simulink model "quarter_sus_imp"  (R2025a)
settings: Solver=FixedStepAuto  StartTime=0.0  StopTime=20  FixedStep=0.001  RelTol=1e-3
model workspace (MAT data in the model file):
  Cs : Simulink.Parameter (value not decoded)
  Cy_f1 = 128915.5
  Cy_r1 = 85943.6
  G0 : Simulink.Parameter (value not decoded)
  IDA_ISD_PBC_bd : Simulink.Parameter (value not decoded)
  IDA_ISD_PBC_c1 : Simulink.Parameter (value not decoded)
  IDA_ISD_PBC_k1 : Simulink.Parameter (value not decoded)
  IDA_ISD_PBC_k2 : Simulink.Parameter (value not decoded)
  IDA_ISD_PBC_r1 : Simulink.Parameter (value not decoded)
  IDA_PBC_cd4 = 2000
  IDA_PBC_kd2 = 10000
  IDA_PBC_r1 = 1.5
  IDA_PBC_r2 = 0.44
  ISD_1_b : Simulink.Parameter (value not decoded)
  ISD_1_c : Simulink.Parameter (value not decoded)
  ISD_1_k1 : Simulink.Parameter (value not decoded)
  ISD_1_k2 : Simulink.Parameter (value not decoded)
  Izz1 = 1536.7
  Ks : Simulink.Parameter (value not decoded)
  Kt : Simulink.Parameter (value not decoded)
  Q : Simulink.Parameter (value not decoded)
  Q_dot : Simulink.Parameter (value not decoded)
  Q_dot_s : Simulink.Parameter (value not decoded)
  Q_dot_u : Simulink.Parameter (value not decoded)
  Q_flec : Simulink.Parameter (value not decoded)
  SHADD_alpha : Simulink.Parameter (value not decoded)
  a1 = 1.015
  a_max : Simulink.Parameter (value not decoded)
  a_min : Simulink.Parameter (value not decoded)
  adva_max : Simulink.Parameter (value not decoded)
  adva_min : Simulink.Parameter (value not decoded)
  as_max : Simulink.Parameter (value not decoded)
  b1 = 1.895
  b_deflec : Simulink.Parameter (value not decoded)
  bump_height : Simulink.Parameter (value not decoded)
  bump_lenth : Simulink.Parameter (value not decoded)
  bump_start : Simulink.Parameter (value not decoded)
  damper_param : Simulink.Parameter (value not decoded)
  deflec_max : Simulink.Parameter (value not decoded)
  done_range : Simulink.Parameter (value not decoded)
  f0 : Simulink.Parameter (value not decoded)
  h1 = 0.54
  imp_Cs : Simulink.Parameter (value not decoded)
  imp_Ks : Simulink.Parameter (value not decoded)
  imp_Ms : Simulink.Parameter (value not decoded)
  inerter_b : Simulink.Parameter (value not decoded)
  inerter_b_2 : Simulink.Parameter (value not decoded)
  inerter_c : Simulink.Parameter (value not decoded)
  inerter_k : Simulink.Parameter (value not decoded)
  inerter_k_2 : Simulink.Parameter (value not decoded)
  ms : Simulink.Parameter (value not decoded)
  mu : Simulink.Parameter (value not decoded)
  noise_seed : Simulink.Parameter (value not decoded)
  punish_Q : Simulink.Parameter (value not decoded)
  punish_R : Simulink.Parameter (value not decoded)
  reward_w_as : Simulink.Parameter (value not decoded)
  reward_w_au : Simulink.Parameter (value not decoded)
  reward_w_defv : Simulink.Parameter (value not decoded)
  road_seed : Simulink.Parameter (value not decoded)
  road_type : Simulink.Parameter (value not decoded)
  sigma_f1 = 0.1
  sigma_r1 = 0.1
  sine_amp : Simulink.Parameter (value not decoded)
  sine_freq : Simulink.Parameter (value not decoded)
  u : Simulink.Parameter (value not decoded)
  vs0 : Simulink.Parameter (value not decoded)
  vu0 : Simulink.Parameter (value not decoded)
  x_max : Simulink.Parameter (value not decoded)
  x_min : Simulink.Parameter (value not decoded)
  xs0 : Simulink.Parameter (value not decoded)
  xu0 : Simulink.Parameter (value not decoded)
symbols that are objects in the model workspace (value not decoded): a_max, a_min, b_deflec, bump_height, bump_lenth, bump_start, Cs, damper_param, f0, G0, IDA_ISD_PBC_bd, IDA_ISD_PBC_c1, IDA_ISD_PBC_k1, IDA_ISD_PBC_k2, IDA_ISD_PBC_r1, imp_Cs, imp_Ks, imp_Ms, Ks, Kt, ms, mu, Q_dot_s, Q_dot_u, Q_flec, road_type, SHADD_alpha, sine_amp, sine_freq, vs0, vu0, xs0, xu0
undefined symbols (not defined in the file or in its folder): ADD, Force, IDA, Imp, PBC, SH, Train, Validation
libraries: fl_lib x32, nesl_utility x27, sdl_lib x2, deeplib x1, simulink x1
(part 4 of 5)

== system quarter_sus_imp/QuarterSuspension /road_profile/origin ==
  Manual Switch : ManualSwitch  CurrentSetting=0
  Radio Button : RadioButtonGroup  LabelPosition=Hide  SelectedLabel=随机路面  ButtonGroupName=Group
  Road_Type : Constant  Value=road_type  OutDataTypeStr=int8
  road_profile : Subsystem
  路面选择 : Constant  Value=3  OutDataTypeStr=int8
  "Road " : Outport
  wires:
  路面选择/1 -> Manual Switch/1
  road_profile/1("Road ") -> "Road "/1  "Zr"
  Manual Switch/1 -> road_profile/1(Road_selection)
  Road_Type/1 -> Manual Switch/2

== system quarter_sus_imp/QuarterSuspension /Subsystem1/Active Suspension/Subsystem ==
  Connection Port : PMIOPort  Side=Left

== system quarter_sus_imp/QuarterSuspension /Subsystem1/Semi Active Air Suspension/Damper ==
  displacement : Inport
  velocity : Inport  Port=2
  current : Inport  Port=3
  Hysteretic : Subsystem  VariantControl=Hysteretic
  Linear : Subsystem  VariantControl=simple linear
  Random Current : Subsystem  VariantControl=Random Current
  semi-active : Subsystem  VariantControl=Semi-active
  simple_Nonlinear : Subsystem  VariantControl=Simple_Nonlinear
  simple_Nonlinear_2d : Subsystem  VariantControl=Simple_Nonlinear_2d
  F_d : Outport
  current_log : Outport  Port=2

== system quarter_sus_imp/QuarterSuspension /Subsystem1/Semi Active Air Suspension/Subsystem ==
  In1 : Inport
  linear : Subsystem  VariantControl=linear
  simple nonlinear : Subsystem  VariantControl=simple nonlinear
  Out1 : Outport

== system quarter_sus_imp/QuarterSuspension /Subsystem1/Semi Active Air Suspension simscape/Damper ==
  displacement : Inport
  velocity : Inport  Port=2
  current : Inport  Port=3
  Hysteretic : Subsystem  VariantControl=Hysteretic
  Random Current : Subsystem  VariantControl=Random Current
  semi-active : Subsystem  VariantControl=Semi-active
  simple_Nonlinear : Subsystem  VariantControl=Simple_Nonlinear
  simple_Nonlinear_2d : Subsystem  VariantControl=Simple_Nonlinear_2d
  F_d : Outport
  current_log : Outport  Port=2

== system quarter_sus_imp/QuarterSuspension /Subsystem1/Semi Active Air Suspension simscape/Subsystem ==
  Connection Port : PMIOPort  Side=Left

== system quarter_sus_imp/QuarterSuspension /Subsystem1/Semi Active Suspension/Damper ==
  displacement : Inport
  velocity : Inport  Port=2
  current : Inport  Port=3
  Hysteretic : Subsystem  VariantControl=Hysteretic
  Random Current : Subsystem  VariantControl=Random Current
  semi-active : Subsystem  VariantControl=Semi-active
  simple_Nonlinear : Subsystem  VariantControl=Simple_Nonlinear
  simple_Nonlinear_2d : Subsystem  VariantControl=Simple_Nonlinear_2d
  F_d : Outport
  current_log : Outport  Port=2

== system quarter_sus_imp/QuarterSuspension /Variant Subsystem/ADD/Subsystem1 ==
  state : Inport
  Demux : Demux  Outputs=11
  Divide : Product  Inputs=**
  Switch1 : Switch  SaturateOnIntegerOverflow=off  InputSameDT=off
  Terminator{,1..6} (7 alike) : Terminator
  c_max : Constant  Value=500
  c_min : Constant  Value=-500
  action : Outport
  wires:
  state/1 -> Demux/1
  Demux/10 -> Terminator2/1
  Demux/7 -> [v_deflection]
  Demux/11 -> Terminator3/1
  Demux/6 -> [deflection]
  Demux/3 -> [as]
  Demux/2 -> [vs]
  Demux/1 -> Terminator6/1
  Demux/5 -> Terminator5/1
  Demux/4 -> Terminator4/1
  Demux/8 -> Terminator/1
  Demux/9 -> Terminator1/1
  c_min/1 -> Switch1/3
  Divide/1 -> Switch1/2
  c_max/1 -> Switch1/1
  [as] -> Divide/1
  [v_deflection] -> Divide/2
  Switch1/1 -> action/1

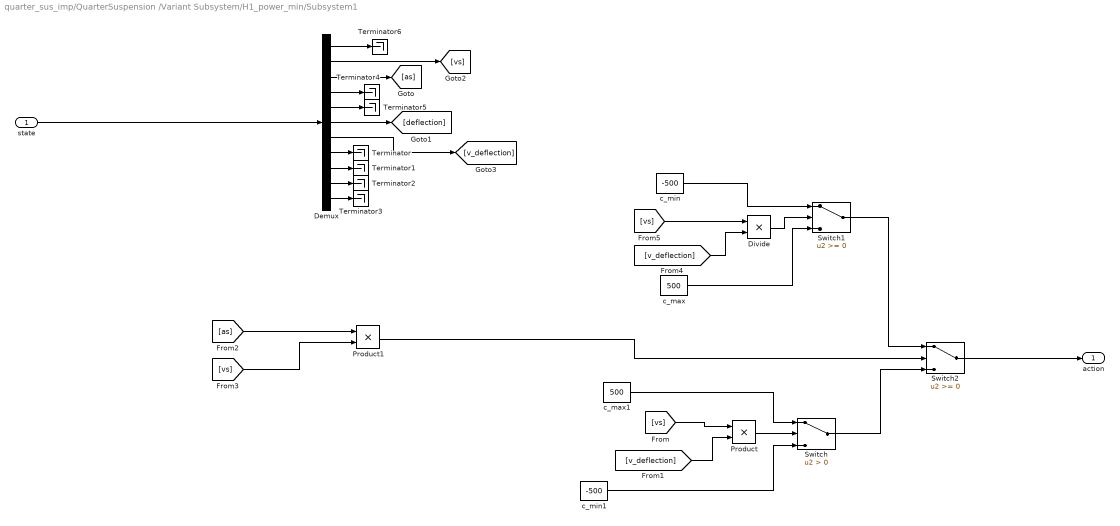
== system quarter_sus_imp/QuarterSuspension /Variant Subsystem/H1_power_min/Subsystem1 ==
  state : Inport
  Demux : Demux  Outputs=11
  Divide : Product  Inputs=**
  Product : Product
  Product1 : Product
  Switch : Switch  Criteria=u2 > Threshold  SaturateOnIntegerOverflow=off  InputSameDT=off
  Switch1 : Switch  SaturateOnIntegerOverflow=off  InputSameDT=off
  Switch2 : Switch  SaturateOnIntegerOverflow=off  InputSameDT=off
  Terminator{,1..6} (7 alike) : Terminator
  c_max : Constant  Value=500
  c_max1 : Constant  Value=500
  c_min : Constant  Value=-500
  c_min1 : Constant  Value=-500
  action : Outport
  wires:
  state/1 -> Demux/1
  Demux/10 -> Terminator2/1
  Demux/7 -> [v_deflection]
  Demux/11 -> Terminator3/1
  Demux/6 -> [deflection]
  Demux/3 -> [as]
  Demux/2 -> [vs]
  Demux/1 -> Terminator6/1
  Demux/5 -> Terminator5/1
  Demux/4 -> Terminator4/1
  Demux/8 -> Terminator/1
  Demux/9 -> Terminator1/1
  c_min/1 -> Switch1/1
  Divide/1 -> Switch1/2
  c_max/1 -> Switch1/3
  [vs] -> Divide/1
  [v_deflection] -> Divide/2
  c_min1/1 -> Switch/3
  Product/1 -> Switch/2
  [v_deflection] -> Product/2
  c_max1/1 -> Switch/1
  [vs] -> Product/1
  [vs] -> Product1/2
  Product1/1 -> Switch2/2
  Switch2/1 -> action/1
  Switch/1 -> Switch2/3
  Switch1/1 -> Switch2/1
  [as] -> Product1/1

== system quarter_sus_imp/QuarterSuspension /Variant Subsystem/IDA-PBC/Subsystem ==
  In1 : Inport
  IDA-PBC 论文控制 : Subsystem  VariantControl=IDAPBC
  IDA_ISD_1号参考控制 : Subsystem  VariantControl=My_IDA_ISD
  我的控制 : Subsystem  VariantControl=MyIDA_PBC
  u : Outport

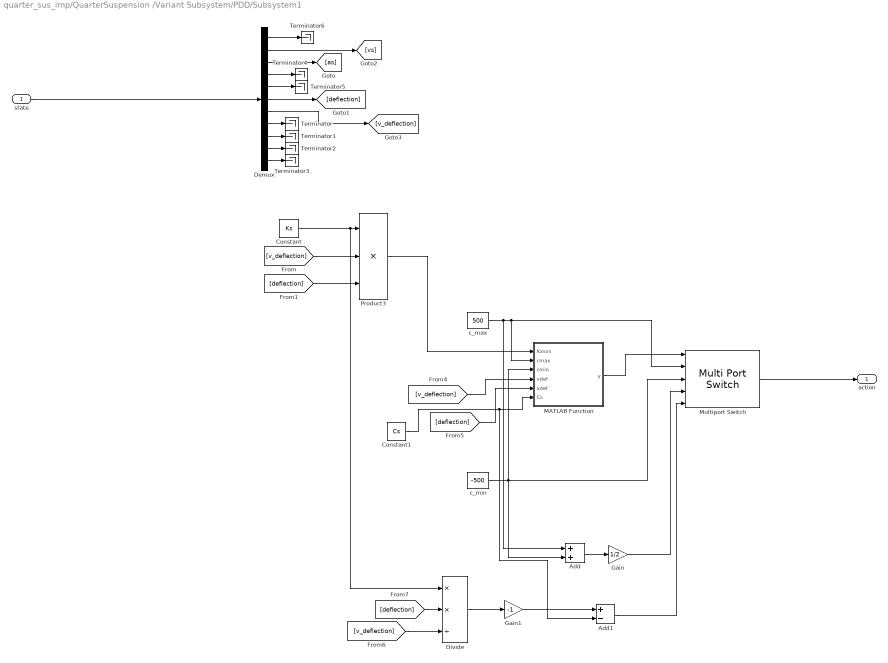
== system quarter_sus_imp/QuarterSuspension /Variant Subsystem/PDD/Subsystem1 ==
  state : Inport
  Add : Sum
  Add1 : Sum  Inputs=+-
  Constant : Constant  Value=Ks
  Constant1 : Constant  Value=Cs
  Demux : Demux  Outputs=11
  Divide : Product  Inputs=**/
  Gain : Gain  Gain=1/2
  Gain1 : Gain  Gain=-1
  MATLAB Function : MATLAB Function  TreatAsAtomicUnit=on
  Multiport Switch : MultiPortSwitch  Inputs=4  SaturateOnIntegerOverflow=off  InputSameDT=off
  Product3 : Product  Inputs=3
  Terminator{,1..6} (7 alike) : Terminator
  c_max : Constant  Value=500
  c_min : Constant  Value=-500
  action : Outport
  wires:
  state/1 -> Demux/1
  Demux/10 -> Terminator2/1
  Demux/7 -> [v_deflection]
  Demux/11 -> Terminator3/1
  Demux/6 -> [deflection]
  Demux/3 -> [as]
  Demux/2 -> [vs]
  Demux/1 -> Terminator6/1
  Demux/5 -> Terminator5/1
  Demux/4 -> Terminator4/1
  Demux/8 -> Terminator/1
  Demux/9 -> Terminator1/1
  c_max/1 -> Multiport Switch/2, MATLAB Function/2(cmax), Add/1
  Multiport Switch/1 -> action/1
  Constant/1 -> Divide/1, Product3/1
  [v_deflection] -> Product3/2
  [deflection] -> Product3/3
  Product3/1 -> MATLAB Function/1(Kxsvs)
  c_min/1 -> Multiport Switch/3, Add/2, MATLAB Function/3(cmin)
  MATLAB Function/1(y) -> Multiport Switch/1
  [v_deflection] -> MATLAB Function/4(vdef)
  Add/1 -> Gain/1
  [deflection] -> MATLAB Function/5(xdef)
  [v_deflection] -> Divide/3
  [deflection] -> Divide/2
  Divide/1 -> Gain1/1
  Gain/1 -> Multiport Switch/4
  Add1/1 -> Multiport Switch/5
  Constant1/1 -> MATLAB Function/6(Cs), Add1/2
  Gain1/1 -> Add1/1

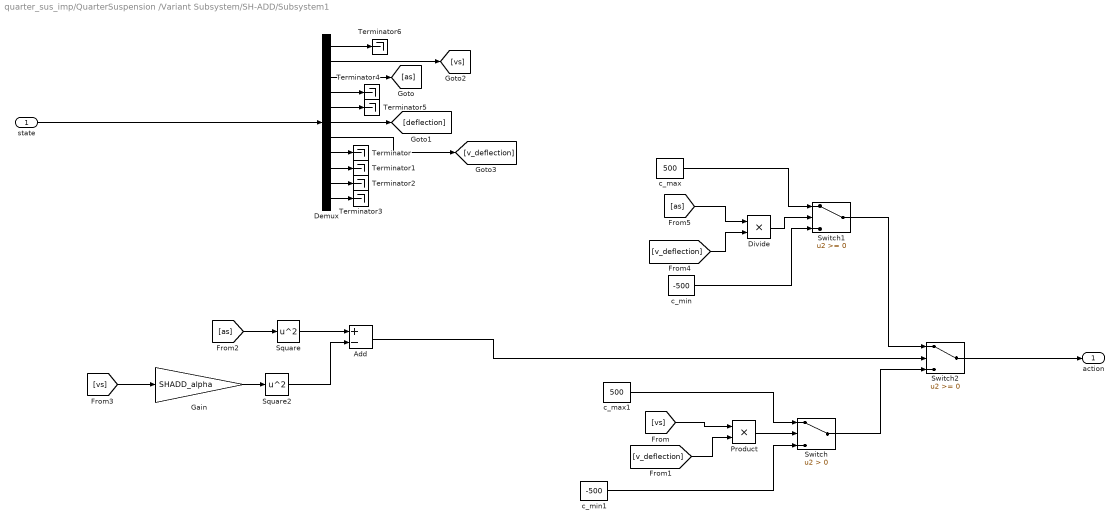
== system quarter_sus_imp/QuarterSuspension /Variant Subsystem/SH-ADD/Subsystem1 ==
  state : Inport
  Add : Sum  Inputs=+-
  Demux : Demux  Outputs=11
  Divide : Product  Inputs=**
  Gain : Gain  Gain=SHADD_alpha
  Product : Product
  Square : Math  Operator=square
  Square2 : Math  Operator=square
  Switch : Switch  Criteria=u2 > Threshold  SaturateOnIntegerOverflow=off  InputSameDT=off
  Switch1 : Switch  SaturateOnIntegerOverflow=off  InputSameDT=off
  Switch2 : Switch  SaturateOnIntegerOverflow=off  InputSameDT=off
  Terminator{,1..6} (7 alike) : Terminator
  c_max : Constant  Value=500
  c_max1 : Constant  Value=500
  c_min : Constant  Value=-500
  c_min1 : Constant  Value=-500
  action : Outport
  wires:
  state/1 -> Demux/1
  Demux/10 -> Terminator2/1
  Demux/7 -> [v_deflection]
  Demux/11 -> Terminator3/1
  Demux/6 -> [deflection]
  Demux/3 -> [as]
  Demux/2 -> [vs]
  Demux/1 -> Terminator6/1
  Demux/5 -> Terminator5/1
  Demux/4 -> Terminator4/1
  Demux/8 -> Terminator/1
  Demux/9 -> Terminator1/1
  c_min/1 -> Switch1/3
  Divide/1 -> Switch1/2
  c_max/1 -> Switch1/1
  [as] -> Divide/1
  [v_deflection] -> Divide/2
  c_min1/1 -> Switch/3
  Product/1 -> Switch/2
  [v_deflection] -> Product/2
  c_max1/1 -> Switch/1
  [vs] -> Product/1
  [as] -> Square/1
  [vs] -> Gain/1
  Square/1 -> Add/1
  Gain/1 -> Square2/1
  Add/1 -> Switch2/2
  Switch2/1 -> action/1
  Switch/1 -> Switch2/3
  Switch1/1 -> Switch2/1
  Square2/1 -> Add/2

== system quarter_sus_imp/QuarterSuspension /Variant Subsystem/Skyhook/Subsystem ==
  In1 : Inport
  Add : Sum  Inputs=+-
  Add1 : Sum  Inputs=+-
  Demux : Demux
  Product : Product
  Switch : Switch  Criteria=u2 > Threshold  SaturateOnIntegerOverflow=off  InputSameDT=off
  c_max : Constant  Value=0.9
  c_min : Constant  Value=0.3
  Out8 : Outport
  wires:
  In1/1 -> Demux/1
  c_min/1 -> Switch/3
  Add1/1 -> [v_deflection]
  Add/1 -> [deflection]
  [vs] -> Product/1
  c_max/1 -> Switch/1
  [v_deflection] -> Product/2
  Product/1 -> Switch/2
  Switch/1 -> Out8/1
  Demux/1 -> Add/1
  Demux/2 -> Add/2
  Demux/3 -> Add1/1
  Demux/4 -> Add1/2

== system quarter_sus_imp/QuarterSuspension /Variant Subsystem/Vaildation-3para-feedback/Impedance Controller ==
  feedback_para : Inport
  est_state : Inport  Port=2
  Add1 : Sum  Inputs=+++
  Demux : Demux  Outputs=3
  Demux2 : Demux  Outputs=5
  Product : Product
  Product2 : Product
  Product3 : Product
  F_imp : Outport
  wires:
  Demux/3 -> [feedback_C]
  Demux/1 -> [feedback_M]
  feedback_para/1 -> Demux/1
  Demux/2 -> [feedback_K]
  est_state/1 -> Demux2/1
  Demux2/1 -> [est_Xs]
  Demux2/2 -> [est_Vs]
  Demux2/4 -> [est_Xdef]
  Demux2/5 -> [est_V_def]
  [est_Vs] -> Product2/2
  [feedback_C] -> Product2/1
  [feedback_K] -> Product3/1
  [est_Xs] -> Product3/2
  Product2/1 -> Add1/1
  Product3/1 -> Add1/2
  Add1/1 -> F_imp/1
  [feedback_M] -> Product/2
  Demux2/3 -> [est_as]
  [est_as] -> Product/1
  Product/1 -> Add1/3

== system quarter_sus_imp/QuarterSuspension /Variant Subsystem/Vaildation-3para-feedback/Subsystem ==
  In1 : Inport
  GOPS_Bridge : Subsystem  VariantControl=GOPS_Bridge
  ONNX : Subsystem  VariantControl=ONNX
  real_act : Outport

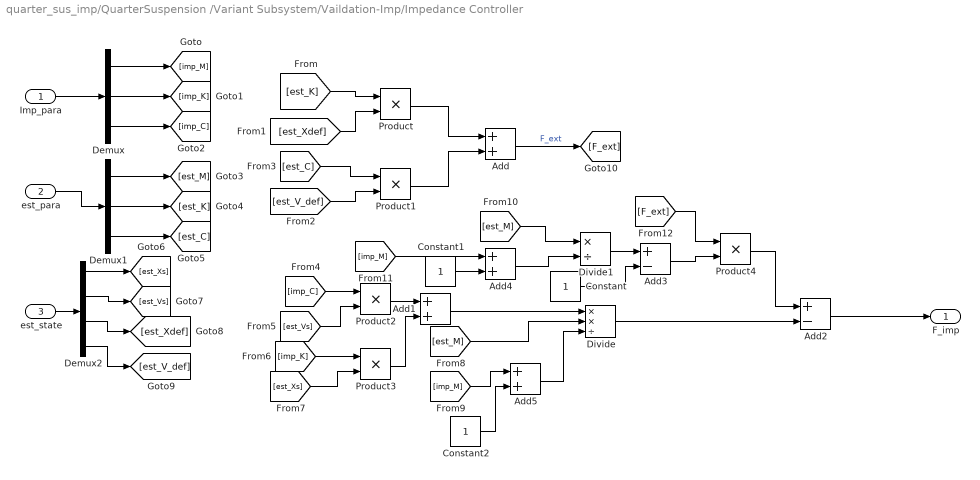
== system quarter_sus_imp/QuarterSuspension /Variant Subsystem/Vaildation-Imp/Impedance Controller ==
  Imp_para : Inport
  est_para : Inport  Port=2
  est_state : Inport  Port=3
  Add{,1,4..5} (4 alike) : Sum
  Add2 : Sum  Inputs=+-
  Add3 : Sum  Inputs=+-
  Constant : Constant
  Constant1 : Constant
  Constant2 : Constant
  Demux : Demux  Outputs=3
  Demux1 : Demux  Outputs=3
  Demux2 : Demux
  Divide : Product  Inputs=**/
  Divide1 : Product  Inputs=*/
  Product{,1..4} (5 alike) : Product
  F_imp : Outport
  wires:
  Demux/3 -> [imp_C]
  Demux/1 -> [imp_M]
  Imp_para/1 -> Demux/1
  Demux/2 -> [imp_K]
  Demux1/1 -> [est_M]
  Demux1/2 -> [est_K]
  est_para/1 -> Demux1/1
  Demux1/3 -> [est_C]
  est_state/1 -> Demux2/1
  Demux2/1 -> [est_Xs]
  Demux2/2 -> [est_Vs]
  Demux2/3 -> [est_Xdef]
  Demux2/4 -> [est_V_def]
  [est_K] -> Product/1
  [est_Xdef] -> Product/2
  [est_C] -> Product1/1
  [est_V_def] -> Product1/2
  Product/1 -> Add/1
  Product1/1 -> Add/2
  Add/1 -> [F_ext]  "F_ext"
  [est_Vs] -> Product2/2
  [imp_C] -> Product2/1
  [imp_K] -> Product3/1
  [est_Xs] -> Product3/2
  Product2/1 -> Add1/1
  Product3/1 -> Add1/2
  Add1/1 -> Divide/1
  [est_M] -> Divide/2
  [imp_M] -> Add5/1
  Divide/1 -> Add2/2
  Add2/1 -> F_imp/1
  [imp_M] -> Add4/1
  [est_M] -> Divide1/1
  Divide1/1 -> Add3/1
  Constant/1 -> Add3/2
  Add3/1 -> Product4/2
  [F_ext] -> Product4/1
  Product4/1 -> Add2/1
  Add4/1 -> Divide1/2
  Constant1/1 -> Add4/2
  Add5/1 -> Divide/3
  Constant2/1 -> Add5/2

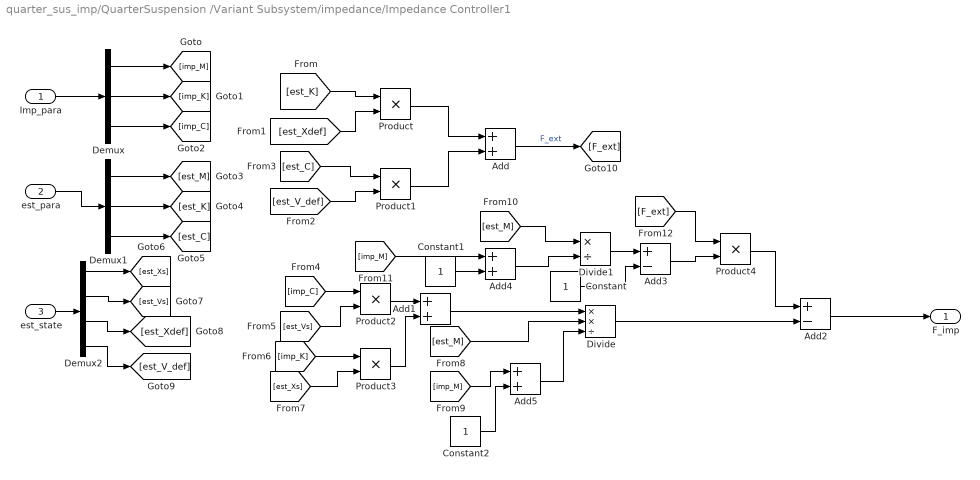
== system quarter_sus_imp/QuarterSuspension /Variant Subsystem/impedance/Impedance Controller1 ==
  Imp_para : Inport
  est_para : Inport  Port=2
  est_state : Inport  Port=3
  Add{,1,4..5} (4 alike) : Sum
  Add2 : Sum  Inputs=+-
  Add3 : Sum  Inputs=+-
  Constant : Constant
  Constant1 : Constant
  Constant2 : Constant
  Demux : Demux  Outputs=3
  Demux1 : Demux  Outputs=3
  Demux2 : Demux
  Divide : Product  Inputs=**/
  Divide1 : Product  Inputs=*/
  Product{,1..4} (5 alike) : Product
  F_imp : Outport
  wires:
  Demux/3 -> [imp_C]
  Demux/1 -> [imp_M]
  Imp_para/1 -> Demux/1
  Demux/2 -> [imp_K]
  Demux1/1 -> [est_M]
  Demux1/2 -> [est_K]
  est_para/1 -> Demux1/1
  Demux1/3 -> [est_C]
  est_state/1 -> Demux2/1
  Demux2/1 -> [est_Xs]
  Demux2/2 -> [est_Vs]
  Demux2/3 -> [est_Xdef]
  Demux2/4 -> [est_V_def]
  [est_K] -> Product/1
  [est_Xdef] -> Product/2
  [est_C] -> Product1/1
  [est_V_def] -> Product1/2
  Product/1 -> Add/1
  Product1/1 -> Add/2
  Add/1 -> [F_ext]  "F_ext"
  [est_Vs] -> Product2/2
  [imp_C] -> Product2/1
  [imp_K] -> Product3/1
  [est_Xs] -> Product3/2
  Product2/1 -> Add1/1
  Product3/1 -> Add1/2
  Add1/1 -> Divide/1
  [est_M] -> Divide/2
  [imp_M] -> Add5/1
  Divide/1 -> Add2/2
  Add2/1 -> F_imp/1
  [imp_M] -> Add4/1
  [est_M] -> Divide1/1
  Divide1/1 -> Add3/1
  Constant/1 -> Add3/2
  Add3/1 -> Product4/2
  [F_ext] -> Product4/1
  Product4/1 -> Add2/1
  Add4/1 -> Divide1/2
  Constant1/1 -> Add4/2
  Add5/1 -> Divide/3
  Constant2/1 -> Add5/2

== system quarter_sus_imp/QuarterSuspension /road_profile/origin/road_profile ==
  note: road selection
      | 1 sine
      | 2 chrip
      | 3 random
      | 4 bump
  Road_selection : Inport  OutDataTypeStr=int8  PortDimensions=1
  Bump : Subsystem
  Multiport Switch : MultiPortSwitch  DataPortOrder=Specify indices  Inputs=4  DataPortIndices={1,2,3,4}  SaturateOnIntegerOverflow=off  InputSameDT=off
  Random : Subsystem
  Scope{,1..3} (4 alike) : Scope
      Scope settings: ActiveDisplayYMinimum=-0.12499  ActiveDisplayYMaximum=0.12499
      Scope1 settings: ActiveDisplayYMinimum=-0.0189  ActiveDisplayYMaximum=0.01881  DataLoggingVariableName=ScopeData2
      Scope2 settings: ActiveDisplayYMinimum=-0.0025  ActiveDisplayYMaximum=0.0225  DataLoggingVariableName=ScopeData3
      Scope3 settings: ActiveDisplayYMinimum=-0.07918  ActiveDisplayYMaximum=0.12812
  Sine Wave : Sin  Amplitude=sine_amp  Frequency=2*pi*sine_freq  SampleTime=0
  chirp : Subsystem
  "Road " : Outport  OutDataTypeStr=double  PortDimensions=1  SampleTime=0  VectorParamsAs1DForOutWhenUnconnected=off
  wires:
  Multiport Switch/1 -> "Road "/1
  Road_selection/1 -> Multiport Switch/1
  chirp/1(Zr) -> Multiport Switch/3, Scope3/1
  Random/1(Zr) -> Scope1/1, Multiport Switch/4
  Sine Wave/1 -> Multiport Switch/2, Scope/1
  Bump/1(Zr) -> Scope2/1, Multiport Switch/5

== system quarter_sus_imp/QuarterSuspension /Subsystem1/Semi Active Air Suspension/Damper/Hysteretic ==
  displacement : Inport
  velocity : Inport  Port=2
  MATLAB Function1 : MATLAB Function  TreatAsAtomicUnit=on
  current : Constant  Value=0.5
  damper_model_param : Constant  Value=[5260.15986746959 -5064.02034514632 2187.37751072939 21338.501498397 -29074.5404615999 8136.94569216912 1627.56191580508 -462.340678729998 -186.716958980886 182.174331735857 172.352642777716 99.5565721972277 -221.254303189626 39.7493031072413 6.28167517189674 0.354804320417945]
  F_d : Outport
  wires:
  damper_model_param/1 -> MATLAB Function1/4(params)
  MATLAB Function1/1(F_d) -> F_d/1
  velocity/1 -> MATLAB Function1/2(velocity)
  displacement/1 -> MATLAB Function1/1(displacement)
  current/1 -> MATLAB Function1/3(I)

== system quarter_sus_imp/QuarterSuspension /Subsystem1/Semi Active Air Suspension/Damper/Linear ==
  velocity : Inport
  Gain : Gain  Gain=Cs
  F_d : Outport
  wires:
  velocity/1 -> Gain/1
  Gain/1 -> F_d/1

== system quarter_sus_imp/QuarterSuspension /Subsystem1/Semi Active Air Suspension/Damper/Random Current ==
  displacement : Inport
  velocity : Inport  Port=2
  MATLAB Function1 : MATLAB Function  TreatAsAtomicUnit=on
  Saturation : Saturate  UpperLimit=1.0  LowerLimit=0
  current : UniformRandomNumber  Minimum=0  SampleTime=0.01
  damper_model_param : Constant  Value=[5260.15986746959 -5064.02034514632 2187.37751072939 21338.501498397 -29074.5404615999 8136.94569216912 1627.56191580508 -462.340678729998 -186.716958980886 182.174331735857 172.352642777716 99.5565721972277 -221.254303189626 39.7493031072413 6.28167517189674 0.354804320417945]
  F_d : Outport
  current_log : Outport  Port=2  SampleTime=0.001
  wires:
  Saturation/1 -> current_log/1, MATLAB Function1/3(I)
  damper_model_param/1 -> MATLAB Function1/4(params)
  MATLAB Function1/1(F_d) -> F_d/1
  velocity/1 -> MATLAB Function1/2(velocity)
  displacement/1 -> MATLAB Function1/1(displacement)
  current/1 -> Saturation/1

== system quarter_sus_imp/QuarterSuspension /Subsystem1/Semi Active Air Suspension/Damper/semi-active ==
  displacement : Inport
  velocity : Inport  Port=2
  current : Inport  Port=3
  MATLAB Function1 : MATLAB Function  TreatAsAtomicUnit=on
  Saturation : Saturate  UpperLimit=1.0  LowerLimit=0
  damper_model_param : Constant  Value=damper_param
  F_d : Outport
  current_log : Outport  Port=2  SampleTime=0.001
  wires:
  current/1 -> Saturation/1
  displacement/1 -> MATLAB Function1/1(displacement)
  velocity/1 -> MATLAB Function1/2(velocity)
  MATLAB Function1/1(F_d) -> F_d/1
  damper_model_param/1 -> MATLAB Function1/4(params)
  Saturation/1 -> MATLAB Function1/3(I), current_log/1

== system quarter_sus_imp/QuarterSuspension /Subsystem1/Semi Active Air Suspension/Damper/simple_Nonlinear ==
  displacement : Inport
  velocity : Inport  Port=2
  1-D Lookup Table : Lookup_n-D  NumberOfTableDimensions=1  BreakpointsForDimension1=[-0.6;-0.5;-0.4;0;0.35;0.45;0.6]  BeginIndexSearchUsingPreviousIndexResult=on  Table=[-700;-680;-600;0;875;960;1020]  InternalRulePriority=Speed  RndMeth=Simplest
  Terminator : Terminator
  F_d : Outport
  wires:
  displacement/1 -> Terminator/1
  velocity/1 -> 1-D Lookup Table/1
  1-D Lookup Table/1 -> F_d/1

== system quarter_sus_imp/QuarterSuspension /Subsystem1/Semi Active Air Suspension/Damper/simple_Nonlinear_2d ==
  displacement : Inport
  velocity : Inport  Port=2
  2-D Lookup Table : Lookup_n-D  BreakpointsForDimension1=[-0.6;-0.15;-0.12;-0.1;0;0.1;0.15;0.2;0.6]  BreakpointsForDimension2=[-0.4;-0.1;0;0.1;0.4]  BeginIndexSearchUsingPreviousIndexResult=on  Table=[-1500 -1500 -1500 -1500 -1500;-1200 -1200 -1200 -1200 -1200;-1100 -1000 -925 -850 -800;-1000 -900 -800 -700 -600;-600 -500 0 600 750;200 150 500 980 1050;1000 900 1075 1090 1150;1700 1700 1700 1700 1700;2700 2700 2700 2700 2700]  InternalRulePriority=Speed  RndMeth=Simplest
      settings: InputPortMap=u0,u1
  F_d : Outport
  wires:
  2-D Lookup Table/1 -> F_d/1
  velocity/1 -> 2-D Lookup Table/1
  displacement/1 -> 2-D Lookup Table/2

== system quarter_sus_imp/QuarterSuspension /Subsystem1/Semi Active Air Suspension/Subsystem/linear ==
  In1 : Inport
  Gain : Gain  Gain=Ks
  Out1 : Outport
  wires:
  In1/1 -> Gain/1
  Gain/1 -> Out1/1

== system quarter_sus_imp/QuarterSuspension /Subsystem1/Semi Active Air Suspension/Subsystem/simple nonlinear ==
  In1 : Inport
  1-D Lookup Table : Lookup_n-D  NumberOfTableDimensions=1  BreakpointsForDimension1=[-0.04,-0.03, -0.02, -0.01, -0.005,-0.004, -0.002,-0.001,0.00, 0.001, 0.002,0.004,0.005,0.01, 0.02,0.03, 0.04]  BeginIndexSearchUsingPreviousIndexResult=on  Table=[-1300,-835,-505,-240,-115,-90,-48,-25,0,10,30,60,80,165,320,435,470]  InternalRulePriority=Speed  RndMeth=Simplest
  Out1 : Outport
  wires:
  1-D Lookup Table/1 -> Out1/1
  In1/1 -> 1-D Lookup Table/1

== system quarter_sus_imp/QuarterSuspension /Subsystem1/Semi Active Air Suspension simscape/Damper/Hysteretic ==
  displacement : Inport
  velocity : Inport  Port=2
  MATLAB Function1 : MATLAB Function  TreatAsAtomicUnit=on
  current : Constant  Value=0.5
  damper_model_param : Constant  Value=[5260.15986746959 -5064.02034514632 2187.37751072939 21338.501498397 -29074.5404615999 8136.94569216912 1627.56191580508 -462.340678729998 -186.716958980886 182.174331735857 172.352642777716 99.5565721972277 -221.254303189626 39.7493031072413 6.28167517189674 0.354804320417945]
  F_d : Outport
  wires:
  current/1 -> MATLAB Function1/3(I)
  displacement/1 -> MATLAB Function1/1(displacement)
  velocity/1 -> MATLAB Function1/2(velocity)
  MATLAB Function1/1(F_d) -> F_d/1
  damper_model_param/1 -> MATLAB Function1/4(params)

== system quarter_sus_imp/QuarterSuspension /Subsystem1/Semi Active Air Suspension simscape/Damper/Random Current ==
  displacement : Inport
  velocity : Inport  Port=2
  MATLAB Function1 : MATLAB Function  TreatAsAtomicUnit=on
  Saturation : Saturate  UpperLimit=1.0  LowerLimit=0
  current : UniformRandomNumber  Minimum=0  SampleTime=0.01
  damper_model_param : Constant  Value=[5260.15986746959 -5064.02034514632 2187.37751072939 21338.501498397 -29074.5404615999 8136.94569216912 1627.56191580508 -462.340678729998 -186.716958980886 182.174331735857 172.352642777716 99.5565721972277 -221.254303189626 39.7493031072413 6.28167517189674 0.354804320417945]
  F_d : Outport
  current_log : Outport  Port=2  SampleTime=0.001
  wires:
  current/1 -> Saturation/1
  displacement/1 -> MATLAB Function1/1(displacement)
  velocity/1 -> MATLAB Function1/2(velocity)
  MATLAB Function1/1(F_d) -> F_d/1
  damper_model_param/1 -> MATLAB Function1/4(params)
  Saturation/1 -> MATLAB Function1/3(I), current_log/1

== system quarter_sus_imp/QuarterSuspension /Subsystem1/Semi Active Air Suspension simscape/Damper/semi-active ==
  displacement : Inport
  velocity : Inport  Port=2
  current : Inport  Port=3
  MATLAB Function1 : MATLAB Function  TreatAsAtomicUnit=on
  Saturation : Saturate  UpperLimit=1.0  LowerLimit=0
  damper_model_param : Constant  Value=[5260.15986746959 -5064.02034514632 2187.37751072939 21338.501498397 -29074.5404615999 8136.94569216912 1627.56191580508 -462.340678729998 -186.716958980886 182.174331735857 172.352642777716 99.5565721972277 -221.254303189626 39.7493031072413 6.28167517189674 0.354804320417945]
  F_d : Outport
  current_log : Outport  Port=2  SampleTime=0.001
  wires:
  Saturation/1 -> current_log/1, MATLAB Function1/3(I)
  damper_model_param/1 -> MATLAB Function1/4(params)
  MATLAB Function1/1(F_d) -> F_d/1
  velocity/1 -> MATLAB Function1/2(velocity)
  displacement/1 -> MATLAB Function1/1(displacement)
  current/1 -> Saturation/1

== system quarter_sus_imp/QuarterSuspension /Subsystem1/Semi Active Air Suspension simscape/Damper/simple_Nonlinear ==
  displacement : Inport
  velocity : Inport  Port=2
  1-D Lookup Table : Lookup_n-D  NumberOfTableDimensions=1  BreakpointsForDimension1=[-0.6;-0.5;-0.4;0;0.35;0.45;0.6]  BeginIndexSearchUsingPreviousIndexResult=on  Table=[-700;-680;-600;0;875;960;1020]  InternalRulePriority=Speed  RndMeth=Simplest
  Terminator : Terminator
  F_d : Outport
  wires:
  1-D Lookup Table/1 -> F_d/1
  velocity/1 -> 1-D Lookup Table/1
  displacement/1 -> Terminator/1

== system quarter_sus_imp/QuarterSuspension /Subsystem1/Semi Active Air Suspension simscape/Damper/simple_Nonlinear_2d ==
  displacement : Inport
  velocity : Inport  Port=2
  2-D Lookup Table : Lookup_n-D  BreakpointsForDimension1=[-0.6;-0.15;-0.12;-0.1;0;0.1;0.15;0.2;0.6]  BreakpointsForDimension2=[-0.4;-0.1;0;0.1;0.4]  BeginIndexSearchUsingPreviousIndexResult=on  Table=[-1500 -1500 -1500 -1500 -1500;-1200 -1200 -1200 -1200 -1200;-1100 -1000 -925 -850 -800;-1000 -900 -800 -700 -600;-600 -500 0 600 750;200 150 500 980 1050;1000 900 1075 1090 1150;1700 1700 1700 1700 1700;2700 2700 2700 2700 2700]  InternalRulePriority=Speed  RndMeth=Simplest
      settings: InputPortMap=u0,u1
  F_d : Outport
  wires:
  displacement/1 -> 2-D Lookup Table/2
  velocity/1 -> 2-D Lookup Table/1
  2-D Lookup Table/1 -> F_d/1

== system quarter_sus_imp/QuarterSuspension /Subsystem1/Semi Active Suspension/Damper/Hysteretic ==
  displacement : Inport
  velocity : Inport  Port=2
  MATLAB Function1 : MATLAB Function  TreatAsAtomicUnit=on
  current : Constant  Value=0.5
  damper_model_param : Constant  Value=[5260.15986746959 -5064.02034514632 2187.37751072939 21338.501498397 -29074.5404615999 8136.94569216912 1627.56191580508 -462.340678729998 -186.716958980886 182.174331735857 172.352642777716 99.5565721972277 -221.254303189626 39.7493031072413 6.28167517189674 0.354804320417945]
  F_d : Outport
  wires:
  current/1 -> MATLAB Function1/3(I)
  displacement/1 -> MATLAB Function1/1(displacement)
  velocity/1 -> MATLAB Function1/2(velocity)
  MATLAB Function1/1(F_d) -> F_d/1
  damper_model_param/1 -> MATLAB Function1/4(params)

== system quarter_sus_imp/QuarterSuspension /Subsystem1/Semi Active Suspension/Damper/Random Current ==
  displacement : Inport
  velocity : Inport  Port=2
  MATLAB Function1 : MATLAB Function  TreatAsAtomicUnit=on
  Saturation : Saturate  UpperLimit=1.0  LowerLimit=0
  current : UniformRandomNumber  Minimum=0  SampleTime=0.01
  damper_model_param : Constant  Value=[5260.15986746959 -5064.02034514632 2187.37751072939 21338.501498397 -29074.5404615999 8136.94569216912 1627.56191580508 -462.340678729998 -186.716958980886 182.174331735857 172.352642777716 99.5565721972277 -221.254303189626 39.7493031072413 6.28167517189674 0.354804320417945]
  F_d : Outport
  current_log : Outport  Port=2  SampleTime=0.001
  wires:
  current/1 -> Saturation/1
  displacement/1 -> MATLAB Function1/1(displacement)
  velocity/1 -> MATLAB Function1/2(velocity)
  MATLAB Function1/1(F_d) -> F_d/1
  damper_model_param/1 -> MATLAB Function1/4(params)
  Saturation/1 -> MATLAB Function1/3(I), current_log/1

== system quarter_sus_imp/QuarterSuspension /Subsystem1/Semi Active Suspension/Damper/semi-active ==
  displacement : Inport
  velocity : Inport  Port=2
  current : Inport  Port=3
  MATLAB Function1 : MATLAB Function  TreatAsAtomicUnit=on
  Saturation : Saturate  UpperLimit=1.0  LowerLimit=0
  damper_model_param : Constant  Value=[5260.15986746959 -5064.02034514632 2187.37751072939 21338.501498397 -29074.5404615999 8136.94569216912 1627.56191580508 -462.340678729998 -186.716958980886 182.174331735857 172.352642777716 99.5565721972277 -221.254303189626 39.7493031072413 6.28167517189674 0.354804320417945]
  F_d : Outport
  current_log : Outport  Port=2  SampleTime=0.001
  wires:
  Saturation/1 -> current_log/1, MATLAB Function1/3(I)
  damper_model_param/1 -> MATLAB Function1/4(params)
  MATLAB Function1/1(F_d) -> F_d/1
  velocity/1 -> MATLAB Function1/2(velocity)
  displacement/1 -> MATLAB Function1/1(displacement)
  current/1 -> Saturation/1

== system quarter_sus_imp/QuarterSuspension /Subsystem1/Semi Active Suspension/Damper/simple_Nonlinear ==
  displacement : Inport
  velocity : Inport  Port=2
  1-D Lookup Table : Lookup_n-D  NumberOfTableDimensions=1  BreakpointsForDimension1=[-0.6;-0.5;-0.4;0;0.35;0.45;0.6]  BeginIndexSearchUsingPreviousIndexResult=on  Table=[-700;-680;-600;0;875;960;1020]  InternalRulePriority=Speed  RndMeth=Simplest
  Terminator : Terminator
  F_d : Outport
  wires:
  1-D Lookup Table/1 -> F_d/1
  velocity/1 -> 1-D Lookup Table/1
  displacement/1 -> Terminator/1

== system quarter_sus_imp/QuarterSuspension /Subsystem1/Semi Active Suspension/Damper/simple_Nonlinear_2d ==
  displacement : Inport
  velocity : Inport  Port=2
  2-D Lookup Table : Lookup_n-D  BreakpointsForDimension1=[-0.6;-0.15;-0.12;-0.1;0;0.1;0.15;0.2;0.6]  BreakpointsForDimension2=[-0.4;-0.1;0;0.1;0.4]  BeginIndexSearchUsingPreviousIndexResult=on  Table=[-1500 -1500 -1500 -1500 -1500;-1200 -1200 -1200 -1200 -1200;-1100 -1000 -925 -850 -800;-1000 -900 -800 -700 -600;-600 -500 0 600 750;200 150 500 980 1050;1000 900 1075 1090 1150;1700 1700 1700 1700 1700;2700 2700 2700 2700 2700]  InternalRulePriority=Speed  RndMeth=Simplest
      settings: InputPortMap=u0,u1
  F_d : Outport
  wires:
  displacement/1 -> 2-D Lookup Table/2
  velocity/1 -> 2-D Lookup Table/1
  2-D Lookup Table/1 -> F_d/1

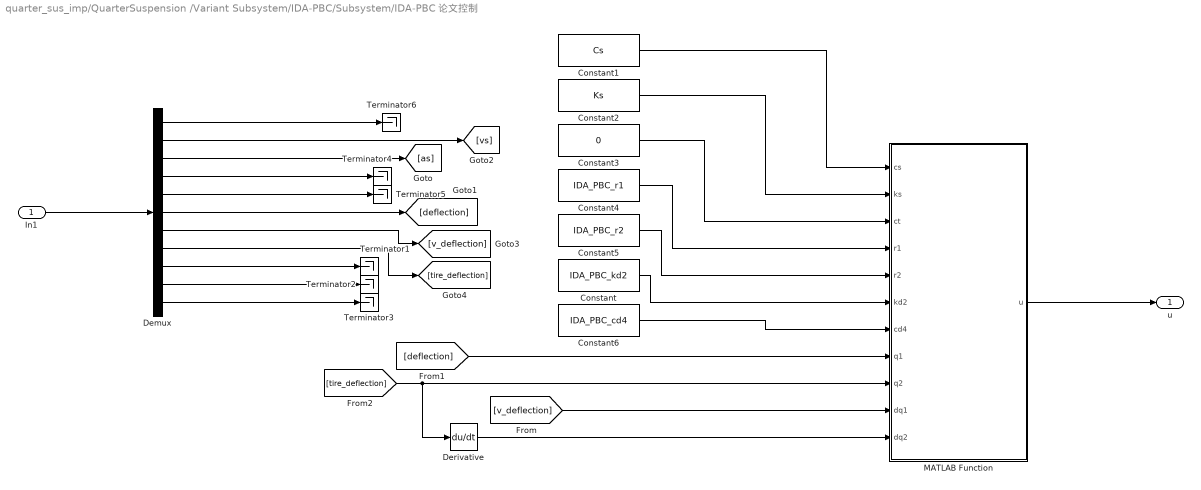
== system quarter_sus_imp/QuarterSuspension /Variant Subsystem/IDA-PBC/Subsystem/IDA-PBC 论文控制 ==
  In1 : Inport
  Constant : Constant  Value=IDA_PBC_kd2
  Constant1 : Constant  Value=Cs
  Constant2 : Constant  Value=Ks
  Constant3 : Constant  Value=0
  Constant4 : Constant  Value=IDA_PBC_r1
  Constant5 : Constant  Value=IDA_PBC_r2
  Constant6 : Constant  Value=IDA_PBC_cd4
  Demux : Demux  Outputs=11
  Derivative : Derivative
  MATLAB Function : MATLAB Function  TreatAsAtomicUnit=on
  Terminator{1..6} (6 alike) : Terminator
  u : Outport
  wires:
  [tire_deflection] -> MATLAB Function/9(q2), Derivative/1
  Demux/8 -> [tire_deflection]
  Demux/10 -> Terminator2/1
  Constant4/1 -> MATLAB Function/4(r1)
  MATLAB Function/1(u) -> u/1
  Demux/11 -> Terminator3/1
  Demux/1 -> Terminator6/1
  Demux/2 -> [vs]
  Constant5/1 -> MATLAB Function/5(r2)
  Demux/3 -> [as]
  Demux/5 -> Terminator5/1
  Derivative/1 -> MATLAB Function/11(dq2)
  Demux/7 -> [v_deflection]
  [v_deflection] -> MATLAB Function/10(dq1)
  Constant/1 -> MATLAB Function/6(kd2)
  [deflection] -> MATLAB Function/8(q1)
  Demux/9 -> Terminator1/1
  In1/1 -> Demux/1
  Constant1/1 -> MATLAB Function/1(cs)
  Constant2/1 -> MATLAB Function/2(ks)
  Constant3/1 -> MATLAB Function/3(ct)
  Demux/4 -> Terminator4/1
  Constant6/1 -> MATLAB Function/7(cd4)
  Demux/6 -> [deflection]

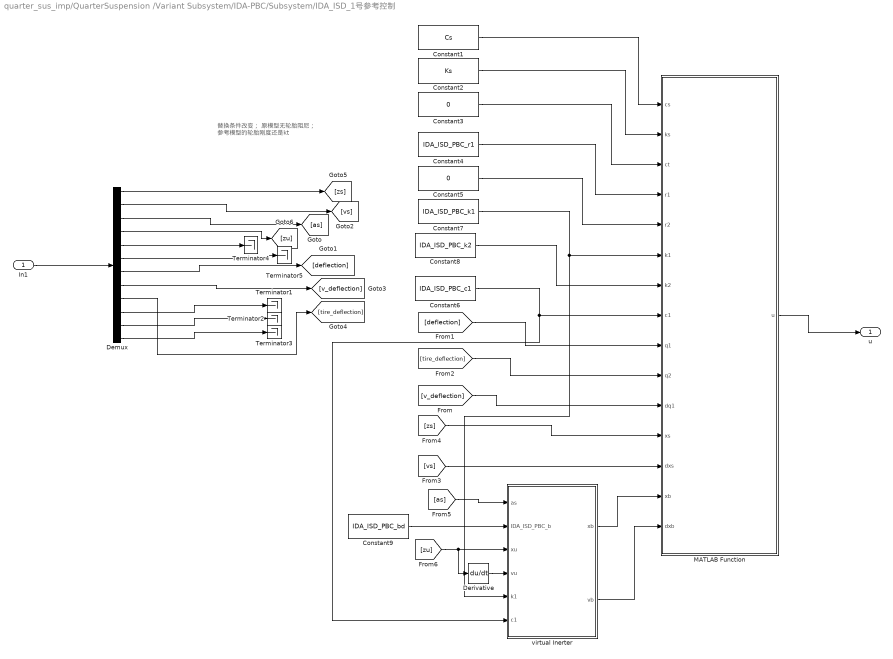
== system quarter_sus_imp/QuarterSuspension /Variant Subsystem/IDA-PBC/Subsystem/IDA_ISD_1号参考控制 ==
  note: 替换条件改变；
      | 原模型无轮胎阻尼；
      | 参考模型的轮胎刚度还是kt
  In1 : Inport
  Constant1 : Constant  Value=Cs
  Constant2 : Constant  Value=Ks
  Constant3 : Constant  Value=0
  Constant4 : Constant  Value=IDA_ISD_PBC_r1
  Constant5 : Constant  Value=0
  Constant6 : Constant  Value=IDA_ISD_PBC_c1
  Constant7 : Constant  Value=IDA_ISD_PBC_k1
  Constant8 : Constant  Value=IDA_ISD_PBC_k2
  Constant9 : Constant  Value=IDA_ISD_PBC_bd
  Demux : Demux  Outputs=12
  Derivative : Derivative
  MATLAB Function : MATLAB Function  TreatAsAtomicUnit=on
  Terminator{1..5} (5 alike) : Terminator
  virtual Inerter : Subsystem
  u : Outport
  wires:
  MATLAB Function/1(u) -> u/1
  [v_deflection] -> MATLAB Function/11(dq1)
  Demux/1 -> [zs]
  Constant4/1 -> MATLAB Function/4(r1)
  [tire_deflection] -> MATLAB Function/10(q2)
  Demux/2 -> [vs]
  Demux/7 -> [deflection]
  Demux/11 -> Terminator2/1
  Constant3/1 -> MATLAB Function/3(ct)
  Demux/12 -> Terminator3/1
  Demux/9 -> [tire_deflection]
  Demux/6 -> Terminator5/1
  Constant5/1 -> MATLAB Function/5(r2)
  Demux/10 -> Terminator1/1
  Constant6/1 -> virtual Inerter/6(c1), MATLAB Function/8(c1)
  Demux/8 -> [v_deflection]
  Constant2/1 -> MATLAB Function/2(ks)
  Demux/3 -> [as]
  Constant1/1 -> MATLAB Function/1(cs)
  [deflection] -> MATLAB Function/9(q1)
  Demux/4 -> [zu]
  In1/1 -> Demux/1
  Constant7/1 -> virtual Inerter/5(k1), MATLAB Function/6(k1)
  Constant8/1 -> MATLAB Function/7(k2)
  [vs] -> MATLAB Function/13(dxs)
  [zs] -> MATLAB Function/12(xs)
  virtual Inerter/1(xb) -> MATLAB Function/14(xb)
  virtual Inerter/2(vb) -> MATLAB Function/15(dxb)
  [as] -> virtual Inerter/1(as)
  [zu] -> Derivative/1, virtual Inerter/3(xu)
  Derivative/1 -> virtual Inerter/4(vu)
  Constant9/1 -> virtual Inerter/2(IDA_ISD_PBC_b)
  Demux/5 -> Terminator4/1

== system quarter_sus_imp/QuarterSuspension /Variant Subsystem/IDA-PBC/Subsystem/我的控制 ==
  note: 替换条件改变；
      | 原模型无轮胎阻尼；
      | 参考模型的轮胎刚度还是kt
  In1 : Inport
  Constant : Constant  Value=IDA_PBC_kd2
  Constant1 : Constant  Value=Cs
  Constant2 : Constant  Value=Ks
  Constant3 : Constant  Value=0
  Constant4 : Constant  Value=IDA_PBC_r1
  Constant5 : Constant  Value=IDA_PBC_r2
  Constant6 : Constant  Value=IDA_PBC_cd4
  Demux : Demux  Outputs=11
  Derivative : Derivative
  MATLAB Function : MATLAB Function  TreatAsAtomicUnit=on
  Terminator{1..6} (6 alike) : Terminator
  u : Outport
  wires:
  Demux/5 -> Terminator5/1
  [v_deflection] -> MATLAB Function/10(dq1)
  Demux/6 -> [deflection]
  [deflection] -> MATLAB Function/8(q1)
  Constant6/1 -> MATLAB Function/7(cd4)
  Constant/1 -> MATLAB Function/6(kd2)
  Demux/4 -> Terminator4/1
  In1/1 -> Demux/1
  Demux/8 -> [tire_deflection]
  Demux/10 -> Terminator2/1
  Constant3/1 -> MATLAB Function/3(ct)
  Demux/9 -> Terminator1/1
  Demux/2 -> [vs]
  Constant2/1 -> MATLAB Function/2(ks)
  Constant1/1 -> MATLAB Function/1(cs)
  Constant5/1 -> MATLAB Function/5(r2)
  Demux/11 -> Terminator3/1
  Demux/3 -> [as]
  Demux/7 -> [v_deflection]
  Demux/1 -> Terminator6/1
  Derivative/1 -> MATLAB Function/11(dq2)
  MATLAB Function/1(u) -> u/1
  Constant4/1 -> MATLAB Function/4(r1)
  [tire_deflection] -> MATLAB Function/9(q2), Derivative/1

== system quarter_sus_imp/QuarterSuspension /Variant Subsystem/Vaildation-3para-feedback/Subsystem/GOPS_Bridge ==
  In1 : Inport
  Level-2 MATLAB S-Function : M-S-Function  FunctionName=gops_validation_bridge  Parameters='D:\Project\GOPS\transform_onnx_network\simu_imp_quartersus\DDPG_231116-155517\network_DDPG_16400_opt.pt'
  actprocess : MATLAB Function  TreatAsAtomicUnit=on  SystemSampleTime=0.001
      settings: MinAlgLoopOccurrences=on
  real_act : Outport
  wires:
  actprocess/1(real_act) -> real_act/1
  Level-2 MATLAB S-Function/1 -> actprocess/1(act)
  In1/1 -> Level-2 MATLAB S-Function/1

== system quarter_sus_imp/QuarterSuspension /Variant Subsystem/Vaildation-3para-feedback/Subsystem/ONNX ==
  In1 : Inport
  Demux : Demux  Outputs=3
  Predict : deeplib/Predict  Network=Network from MAT-file  NetworkFunction=squeezenet  NetworkFilePath=D:\Project\GOPS\gops\env\env_matlab\resources\simu_quartersuspension\DDPG-3para1-onnx.mat  MiniBatchSize=1  InputDataFormats={'',''}  Predictions=on  Activations={}  ForceInterpretedSim=off  EnableDLNetwork=on
  Reshape : Reshape  OutputDimensionality=Row vector (2-D)
  Vector Concatenate : Concatenate  NumInputs=3
  real_act : Outport
  wires:
  Vector Concatenate/1 -> Reshape/1
  Reshape/1 -> Predict/1
  Predict/1 -> real_act/1
  Demux/2 -> Vector Concatenate/2
  In1/1 -> Demux/1
  Demux/3 -> Vector Concatenate/3
  Demux/1 -> Vector Concatenate/1

== system quarter_sus_imp/QuarterSuspension /road_profile/origin/road_profile/Bump ==
  Add : Sum
  Add1 : Sum  Inputs=+-
  Clock1 : Clock
  Constant : Constant  Value=bump_height
  Constant1 : Constant  Value=0
  Constant2 : Constant  Value=u
  Constant3 : Constant  Value=bump_start
  Constant4 : Constant  Value=bump_lenth
  Divide : Product  Inputs=*/
  Gain : Gain  Gain=1/3.6
  Product : Product
  Sine Wave1 : Sin  TimeSource=Use external signal  Amplitude=bump_height  Frequency=2*pi*1  Phase=-1/2*pi  SampleTime=0
  Switch : Switch  Criteria=u2 > Threshold  Threshold=bump_start  SaturateOnIntegerOverflow=off  InputSameDT=off
  Switch1 : Switch  Criteria=u2 > Threshold  Threshold=bump_lenth+bump_start  SaturateOnIntegerOverflow=off  InputSameDT=off
  Zr : Outport  VectorParamsAs1DForOutWhenUnconnected=off
  wires:
  Divide/1 -> Sine Wave1/1
  Constant/1 -> Add/2
  Add/1 -> Switch/1
  Constant4/1 -> Divide/2
  Add1/1 -> Divide/1
  Product/1 -> Gain/1
  Constant2/1 -> Product/1
  Constant3/1 -> Add1/2
  Constant1/1 -> Switch1/1, Switch/3
  Switch/1 -> Switch1/3
  Gain/1 -> Switch1/2, Switch/2, Add1/1
  Sine Wave1/1 -> Add/1
  Clock1/1 -> Product/2
  Switch1/1 -> Zr/1

== system quarter_sus_imp/QuarterSuspension /road_profile/origin/road_profile/Random ==
  Add : Sum
  Gain : Gain  Gain=2*pi*sqrt(G0*u)
  Gain1 : Gain  Gain=-2*pi*f0
  Integrator : Integrator
  WhiteNoise : simulink/Sources/Band-Limited White Noise  Cov=[0.0005]  Ts=0.01  seed=[114514]
  Zr : Outport  VectorParamsAs1DForOutWhenUnconnected=off
  wires:
  Integrator/1 -> Zr/1, Gain1/1
  Gain1/1 -> Add/2
  Add/1 -> Integrator/1
  Gain/1 -> Add/1
  WhiteNoise/1 -> Gain/1

== system quarter_sus_imp/QuarterSuspension /road_profile/origin/road_profile/chirp ==
  note: 幅值
  note: 30hz
  note: f=t*0.2
  note: Frequency=0.2*t [Hz]
  note: x=sin(0.2*pi*t*t)/(0.2*pi*t)
  Clock1 : Clock
  Constant1 : Constant  Value=0.001  SampleTime=0.001
  Constant2 : Constant
  Constant3 : Constant  Value=pi  SampleTime=0.001
  Divide4 : Product  Inputs=*/
  Divide5 : Product  Inputs=**
  Divide6 : Product  Inputs=**
  Divide7 : Product  Inputs=**
  Gain1 : Gain  Gain=0.1
  Gain3 : Gain  Gain=0.4
  Math Function2 : Math  Operator=square  SignedPower=on
  Switch : Switch  Criteria=u2 > Threshold  SaturateOnIntegerOverflow=off  InputSameDT=off
  Trigonometric Function1 : Trigonometry
  Zr : Outport  VectorParamsAs1DForOutWhenUnconnected=off
  wires:
  Constant2/1 -> Divide4/1
  Switch/1 -> Divide5/1, Math Function2/1
  Divide5/1 -> Divide4/2
  Divide4/1 -> Divide6/1
  Trigonometric Function1/1 -> Divide6/2
  Divide7/1 -> Trigonometric Function1/1
  Math Function2/1 -> Divide7/1
  Constant3/1 -> Gain3/1
  Gain3/1 -> Divide5/2, Divide7/2
  Divide6/1 -> Gain1/1
  Clock1/1 -> Switch/2, Switch/1
  Constant1/1 -> Switch/3
  Gain1/1 -> Zr/1

== system quarter_sus_imp/QuarterSuspension /Variant Subsystem/IDA-PBC/Subsystem/IDA_ISD_1号参考控制/virtual Inerter ==
  as : Inport
  IDA_ISD_PBC_b : Inport  Port=2
  xu : Inport  Port=3
  vu : Inport  Port=4
  k1 : Inport  Port=5
  c1 : Inport  Port=6
  Integrator : Integrator
  Integrator1 : Integrator
  MATLAB Function : MATLAB Function  TreatAsAtomicUnit=on
  Memory : Memory
  Memory1 : Memory
  xb : Outport
  vb : Outport  Port=2
  wires:
  Integrator/1 -> Memory/1, vb/1, Integrator1/1  "vb"
  MATLAB Function/1(y) -> Integrator/1  "ab"
  Integrator1/1 -> Memory1/1, xb/1  "xb"
  IDA_ISD_PBC_b/1 -> MATLAB Function/8(bd)
  as/1 -> MATLAB Function/1(as)
  Memory/1 -> MATLAB Function/5(vb)
  Memory1/1 -> MATLAB Function/4(xb)
  xu/1 -> MATLAB Function/2(xu)
  vu/1 -> MATLAB Function/3(vu)
  k1/1 -> MATLAB Function/6(k1)
  c1/1 -> MATLAB Function/7(c1)

== matlab function quarter_sus_imp/QuarterSuspension /Variant Subsystem/IDA-PBC/Subsystem/IDA-PBC 论文控制/MATLAB Function ==
  data: cs input; ks input; ct input; r1 input; u output; r2 input; kd2 input; cd4 input; q1 input; q2 input; dq1 input; dq2 input
function u = calculateEquation(cs, ks,ct, r1, r2, kd2,cd4, q1,q2,dq1,dq2)
    % Calculate each term of the equation
    term1 = (ks - r2*kd2)*q1;
    term2 = (r1 - r2)*kd2*q2 + cs*dq1;
    term4 = r2 * (r2 - r1)* cd4;
    term3 = ((r1*r2*(r2 - 2)*ct +term4)*dq1) / (r1 - r2)^2;
    
    term5 = (ct*r1*r2 / (r1 - r2) - cd4) * dq2;

    % Sum all terms to get u
    u = term1 + term2 + term3 - term5;
end

== matlab function quarter_sus_imp/QuarterSuspension /Subsystem1/Semi Active Suspension/Damper/Hysteretic/MATLAB Function1 ==
  data: displacement input; F_d output; velocity input; I input; params input
function F_d = improvedHystereticModel(displacement, velocity, I, params)
    % 从params数组中提取模型参数
    c1 = params(1); c2 = params(2); c3 = params(3);
    k1 = params(4); k2 = params(5); k3 = params(6);
    alpha1 = params(7); alpha2 = params(8);
    % f01 = params(9); f02 = params(10); f03 = params(11); % 这些参数似乎在模型中未使用
    gamma1 = params(12); gamma2 = params(13); gamma3 = params(14);
    beta = params(15); delta = params(16);

    % 根据I计算c, k, alpha, 和 gamma
    c = c1 * I^2 + c2 * I + c3;
    k = k1 * I^2 + k2 * I + k3;
    alpha = alpha1 * I + alpha2;
    gamma = gamma1 * I^2 + gamma2 * I + gamma3;

    % 计算c^*和z
    c_star = gamma * (sign(velocity) + 1);
    z = tanh(beta * velocity + delta * sign(displacement));

    % 计算减震器力
    F_d = (c + c_star) * velocity + k * displacement + alpha * z;
end

== matlab function quarter_sus_imp/QuarterSuspension /Subsystem1/Semi Active Suspension/Damper/Random Current/MATLAB Function1 ==
  data: displacement input; F_d output; velocity input; I input; params input
function F_d = improvedHystereticModel(displacement, velocity, I, params)
    % 从params数组中提取模型参数
    c1 = params(1); c2 = params(2); c3 = params(3);
    k1 = params(4); k2 = params(5); k3 = params(6);
    alpha1 = params(7); alpha2 = params(8);
    % f01 = params(9); f02 = params(10); f03 = params(11); % 这些参数似乎在模型中未使用
    gamma1 = params(12); gamma2 = params(13); gamma3 = params(14);
    beta = params(15); delta = params(16);

    % 根据I计算c, k, alpha, 和 gamma
    c = c1 * I^2 + c2 * I + c3;
    k = k1 * I^2 + k2 * I + k3;
    alpha = alpha1 * I + alpha2;
    gamma = gamma1 * I^2 + gamma2 * I + gamma3;

    % 计算c^*和z
    c_star = gamma * (sign(velocity) + 1);
    z = tanh(beta * velocity + delta * sign(displacement));

    % 计算减震器力
    F_d = (c + c_star) * velocity + k * displacement + alpha * z;
end

== matlab function quarter_sus_imp/QuarterSuspension /Subsystem1/Semi Active Suspension/Damper/semi-active/MATLAB Function1 ==
  data: displacement input; F_d output; velocity input; I input; params input
function F_d = improvedHystereticModel(displacement, velocity, I, params)
    % 从params数组中提取模型参数
    c1 = params(1); c2 = params(2); c3 = params(3);
    k1 = params(4); k2 = params(5); k3 = params(6);
    alpha1 = params(7); alpha2 = params(8);
    % f01 = params(9); f02 = params(10); f03 = params(11); % 这些参数似乎在模型中未使用
    gamma1 = params(12); gamma2 = params(13); gamma3 = params(14);
    beta = params(15); delta = params(16);

    % 根据I计算c, k, alpha, 和 gamma
    c = c1 * I^2 + c2 * I + c3;
    k = k1 * I^2 + k2 * I + k3;
    alpha = alpha1 * I + alpha2;
    gamma = gamma1 * I^2 + gamma2 * I + gamma3;

    % 计算c^*和z
    c_star = gamma * (sign(velocity) + 1);
    z = tanh(beta * velocity + delta * sign(displacement));

    % 计算减震器力
    F_d = (c + c_star) * velocity + k * displacement + alpha * z;
end

== matlab function quarter_sus_imp/QuarterSuspension /Variant Subsystem/IDA-PBC/Subsystem/IDA_ISD_1号参考控制/MATLAB Function ==
  data: cs input; ks input; ct input; r1 input; u output; r2 input; k1 input; k2 input; c1 input; q1 input; q2 input; dq1 input; xs input; dxs input; xb input; dxb input
function u = calculateEquation(cs, ks,ct, r1, r2,k1, k2,c1, q1,q2,dq1,xs,dxs,xb,dxb)
    % Calculate each term of the equation
  
    term1 = ks*q1;
    term2 = (cs+c1)*dq1;

    term4 = -k2*(xs-xb)/r1;

    term3 = -k1*q2/r1;
    
    term5 = -c1*(dxs-dxb);

    % Sum all terms to get u
    u = term1 + term2 + term3 +term4+ term5;
end

== matlab function quarter_sus_imp/QuarterSuspension /Variant Subsystem/IDA-PBC/Subsystem/IDA_ISD_1号参考控制/virtual Inerter/MATLAB Function ==
  data: as input; y output; xu input; vu input; xb input; vb input; k1 input; c1 input; bd input
function y = fcn(as,xu,vu,xb,vb,k1,c1,bd)

y = as-(k1*(xb-xu)+c1*(vb-vu))/bd;

== matlab function quarter_sus_imp/QuarterSuspension /Subsystem1/Semi Active Air Suspension simscape/Damper/Hysteretic/MATLAB Function1 ==
  data: displacement input; F_d output; velocity input; I input; params input
function F_d = improvedHystereticModel(displacement, velocity, I, params)
    % 从params数组中提取模型参数
    c1 = params(1); c2 = params(2); c3 = params(3);
    k1 = params(4); k2 = params(5); k3 = params(6);
    alpha1 = params(7); alpha2 = params(8);
    % f01 = params(9); f02 = params(10); f03 = params(11); % 这些参数似乎在模型中未使用
    gamma1 = params(12); gamma2 = params(13); gamma3 = params(14);
    beta = params(15); delta = params(16);

    % 根据I计算c, k, alpha, 和 gamma
    c = c1 * I^2 + c2 * I + c3;
    k = k1 * I^2 + k2 * I + k3;
    alpha = alpha1 * I + alpha2;
    gamma = gamma1 * I^2 + gamma2 * I + gamma3;

    % 计算c^*和z
    c_star = gamma * (sign(velocity) + 1);
    z = tanh(beta * velocity + delta * sign(displacement));

    % 计算减震器力
    F_d = (c + c_star) * velocity + k * displacement + alpha * z;
end

== matlab function quarter_sus_imp/QuarterSuspension /Subsystem1/Semi Active Air Suspension simscape/Damper/Random Current/MATLAB Function1 ==
  data: displacement input; F_d output; velocity input; I input; params input
function F_d = improvedHystereticModel(displacement, velocity, I, params)
    % 从params数组中提取模型参数
    c1 = params(1); c2 = params(2); c3 = params(3);
    k1 = params(4); k2 = params(5); k3 = params(6);
    alpha1 = params(7); alpha2 = params(8);
    % f01 = params(9); f02 = params(10); f03 = params(11); % 这些参数似乎在模型中未使用
    gamma1 = params(12); gamma2 = params(13); gamma3 = params(14);
    beta = params(15); delta = params(16);

    % 根据I计算c, k, alpha, 和 gamma
    c = c1 * I^2 + c2 * I + c3;
    k = k1 * I^2 + k2 * I + k3;
    alpha = alpha1 * I + alpha2;
    gamma = gamma1 * I^2 + gamma2 * I + gamma3;

    % 计算c^*和z
    c_star = gamma * (sign(velocity) + 1);
    z = tanh(beta * velocity + delta * sign(displacement));

    % 计算减震器力
    F_d = (c + c_star) * velocity + k * displacement + alpha * z;
end

== matlab function quarter_sus_imp/QuarterSuspension /Subsystem1/Semi Active Air Suspension simscape/Damper/semi-active/MATLAB Function1 ==
  data: displacement input; F_d output; velocity input; I input; params input
function F_d = improvedHystereticModel(displacement, velocity, I, params)
    % 从params数组中提取模型参数
    c1 = params(1); c2 = params(2); c3 = params(3);
    k1 = params(4); k2 = params(5); k3 = params(6);
    alpha1 = params(7); alpha2 = params(8);
    % f01 = params(9); f02 = params(10); f03 = params(11); % 这些参数似乎在模型中未使用
    gamma1 = params(12); gamma2 = params(13); gamma3 = params(14);
    beta = params(15); delta = params(16);

    % 根据I计算c, k, alpha, 和 gamma
    c = c1 * I^2 + c2 * I + c3;
    k = k1 * I^2 + k2 * I + k3;
    alpha = alpha1 * I + alpha2;
    gamma = gamma1 * I^2 + gamma2 * I + gamma3;

    % 计算c^*和z
    c_star = gamma * (sign(velocity) + 1);
    z = tanh(beta * velocity + delta * sign(displacement));

    % 计算减震器力
    F_d = (c + c_star) * velocity + k * displacement + alpha * z;
end

== matlab function quarter_sus_imp/QuarterSuspension /reward_cal/cal_reward ==
  data: state_deflec input; b_def input; reward output; Q_flec input
function reward = fun_reward(state_deflec,b_def,Q_flec)

if state_deflec^2 - b_def^2 > -0.0002
    r_dflec = 1000;
else
    r_dflec = 1/2*log(b_def^2/(b_def^2-state_deflec^2));%定义动行程的BLF函数
end
% Q_r = blkdiag(Q,Q_dot);
% state_r  = [state_deflec,acc];
% reward = state * Q * state'+acc * Q_dot * acc'; %简单二次型reward 考虑加速度与四个状态
% reward  = state_r * Q_r * state_r'; %简单二次型 考虑加速度和动行程
reward = r_dflec * Q_flec; % 二次型加BLF组合
